simulink model "sm_tVtest_chain_trackSeg"  (R2026a)
settings: Solver=ode23t  AbsTol=1e-3  EnableMultiTasking=on
undefined symbols (not defined in the file): Excv, ExcvI2R4, X, Y, Z
libraries: sm_lib x13, sm_trackV_lib_chain_segment x12, nesl_utility x1
Description:
  | Excavator Track Segments
  | Copyright 2023-2026 The MathWorks, Inc.
settings Model: Creator=smiller  LastModifiedBy=smiller
settings DebuggingCC: SubsystemReferenceDiagnosticForUnitTest=warning
settings SimscapeCC: SimscapeNominalValues="[{\"value\":\"1\",\"unit\":\"A\"},{\"value\":\"1\",\"unit\":\"bar\"},{\"value\":\"1\",\"unit\":\"cm^2\"},{\"value\":\"1\",\"unit\":\"cm^3/s\"},{\"value\":\"1\",\"unit\":\"kJ/kg\"},{\"value\":\"1\",\"unit\":\"kW\"},{\"value\":\"1\",\"unit\":\"l\"},{\"value\":\"1\",\"unit\":\"N\"},{\"value\":\"1\",\"unit\":\"N*m\"},{\"value\":\"1\",\"unit\":\"V\"}]"  SimscapeLogSimulationStatistics=on
settings ExplorerConfigSet: InternalSimMechanicsExplorerSettings="<ExplorerConfiguration><canonicalview>default</canonicalview><AnimationSetting><BasePlaybackSpeed>1.0</BasePlaybackSpeed><PlaybackSpeedFactor>1.0</PlaybackSpeedFactor></AnimationSetting><TilePanel><TileInfo><Tiles Columns=\"1\" Count=\"1\" Rows=\"1\"><Column Weight=\"1\"/><Row Weight=\"1\"/><Tile Height=\"1\" Width=\"1\" X=\"0\" Y=\"0\"/></Tiles></TileInfo><SceneInfo><SceneViewer><BGColor><R>1</R><G>1</G><B>1</B></BGColor><Camera><DoPerspective>off</DoPerspective><Position><X>0.602162155298437085</X><Y>-1.48336517440419313</Y><Z>-12.2297850923587443</Z></Position><Center><X>-0.207049076284216343</X><Y>-0.366682176808429294</Y><Z>0.0032695390144664941</Z></Center><Up><X>0.00405979016857013243</X><Y>0.995875537710112058</Y><Z>-0.0906390175056120545</Z></Up><ViewLimDist>1</ViewLimDist><YLim>0.528639925542969458</YLim><XLim>0.496349528694795095</XLim></Camera></SceneViewer></SceneInfo></TilePanel><MechEditorPanel><Cameras/><GfxPanelCameraMap/><VideoCreator><PlaybackSpeedRatio>1.0</PlaybackSpeedRatio><FrameRate>30</FrameRate><VideoFormat>Motion JPEG AVI</VideoFormat><FrameSize>auto</FrameSize></VideoCreator></MechEditorPanel></ExplorerConfiguration>"

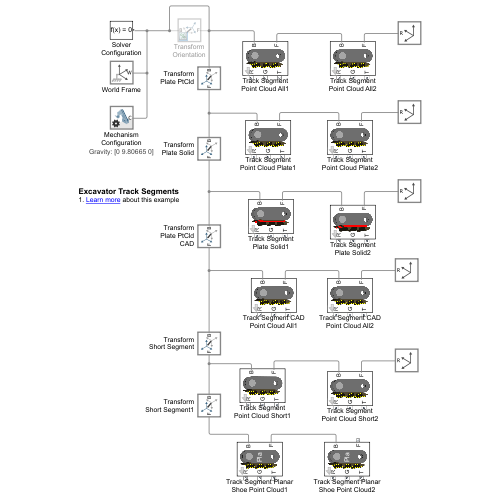
[thumbnail: Simulink's stored preview of the top-level diagram]
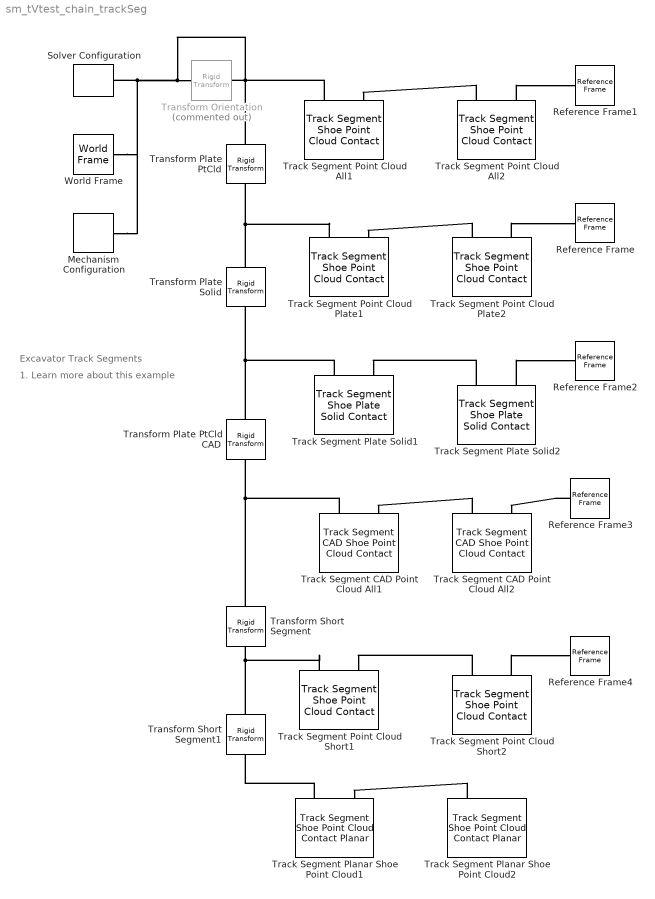
== system sm_tVtest_chain_trackSeg ==
  note: Excavator Track Segments
  note: 1. Learn more about this example
  Mechanism Configuration : sm_lib/Utilities/Mechanism Configuration  UniformGravity=Constant  GravityVector=[0 9.80665 0]  GravityVectorUnits=m/s^2  LinearizationDelta=0.001  JointModeTransitionNonlinearIterations=2
      settings: AttributesFormatString=Gravity: %<GravityVector>
  Reference Frame{,1..4} (5 alike) : sm_lib/Frames and Transforms/Reference Frame
  Solver Configuration : nesl_utility/Solver Configuration  PhysicalDomain=network_engine_domain  SubClassName=solver  LeftPortType=input  RightPortType=generic  Tones=[]  Harmonics=[]  SimulateNoise=off  Profile=off  UseLocalSampling=off  EnableSwitchedLinearOptims=on  FrequencyDomain=off  UseCCode=off  RelTol=0.001  AbsTol=1e-06  MinStep=1e-09  ToWorkspace=off  RevertToSquareIcSolve=off  NumHomotopyIterations=100  PhasorMode=off  PhasorModeNumHarmonics=1  ConsistencySolver=NEWTON_XTOL_AFTER_FTOL  CanonicalOrdering=UNORDERED  OptimizeIntermediates=UNOPTIMIZED  IndexReductionMethod=DerivativeReplacement  DoDC=off  ResidualTolerance=1e-09  ConsistencyTolSource=GLOBAL  ConsistencyAbsTol=0.001  ConsistencyRelTol=0.001  ConsistencyTolFactor=0.001  UseLocalSolver=off  LocalSolverChoice=NE_BACKWARD_EULER_ADVANCER  ResolveIndetEquations=on  FunctionEvalNumThread=1  LocalSolverSampleTime=0.001  DoFixedCost=off  MaxNonlinIter=3  MaxModeIter=2  ComputeImpulses=off  ImpulseIterations=2  LinearAlgebra=Sparse  LinearAlgebraNumThread=0  EquationFormulation=NE_TIME_EF  DelaysMemoryBudget=1024  AutomaticFiltering=on  FilteringTimeConstant=0.001  PartitionStorageMethod=AS_NEEDED  PartitionMemoryBudget=1024  PartitionMethod=FAST  MultibodyUseLocalSolver=off  MultibodyLocalSolverChoice=ODE1  MultibodyLocalSolverSampleTime=0.001
  Track Segment Plate Solid1 : sm_trackV_lib_chain_segment/Track Segment Shoe Plate Solid Contact  chain_wid=Excv.Chain.chain_wid  chain_seg_m=Excv.Chain.link_m  chain_seg_cg=Excv.Chain.link_cg  chain_seg_moi=Excv.Chain.link_moi  chain_seg_poi=Excv.Chain.link_poi  plate_h=Excv.Chain.plate_h  plate_xc=Excv.Chain.plate_xc  plate_thk=Excv.Chain.plate_thk  pin_sep=Excv.Chain.pin_sep  plate_ang=Excv.Chain.plate_ang  plate_clr=Excv.Chain.plate_clr  plate_opc=Excv.Chain.plate_opc  pin_len=Excv.Chain.pin_len  pin_rad=Excv.Chain.pin_rad  pin_clr=Excv.Chain.pin_clr  pin_opc=Excv.Chain.pin_opc  shoe_xc=Excv.Shoe.xc  shoe_w=Excv.Shoe.w  shoe_m=Excv.Shoe.mass  shoe_cg=Excv.Shoe.cg  shoe_moi=Excv.Shoe.moi  shoe_poi=Excv.Shoe.poi  shoe_clr=Excv.Shoe.clr  shoe_opc=Excv.Shoe.opc  posTgtSpecify=on  posTgtPriority=High  PositionTargetValue=0  DampingCoefficient=1.0  shoe_plate_h=Excv.Shoe.pad_h  shoe_plate_l=Excv.Shoe.l  shoe_plate_contact_clr=Excv.Shoe.ground_contact.plate_solid.clr  shoe_plate_contact_opc=Excv.Shoe.ground_contact.plate_solid.opc*0+1  chain_to_roller_clr=Excv.Chain.roller_contact.clr  chain_to_roller_opc=Excv.Chain.roller_contact.opc  chain_to_teeth_clr=Excv.Chain.teeth_contact.clr  chain_to_teeth_opc=Excv.Chain.teeth_contact.opc
  Track Segment Plate Solid2 : sm_trackV_lib_chain_segment/Track Segment Shoe Plate Solid Contact  chain_wid=Excv.Chain.chain_wid  chain_seg_m=Excv.Chain.link_m  chain_seg_cg=Excv.Chain.link_cg  chain_seg_moi=Excv.Chain.link_moi  chain_seg_poi=Excv.Chain.link_poi  plate_h=Excv.Chain.plate_h  plate_xc=Excv.Chain.plate_xc  plate_thk=Excv.Chain.plate_thk  pin_sep=Excv.Chain.pin_sep  plate_ang=Excv.Chain.plate_ang  plate_clr=Excv.Chain.plate_clr  plate_opc=Excv.Chain.plate_opc  pin_len=Excv.Chain.pin_len  pin_rad=Excv.Chain.pin_rad  pin_clr=Excv.Chain.pin_clr  pin_opc=Excv.Chain.pin_opc  shoe_xc=Excv.Shoe.xc  shoe_w=Excv.Shoe.w  shoe_m=Excv.Shoe.mass  shoe_cg=Excv.Shoe.cg  shoe_moi=Excv.Shoe.moi  shoe_poi=Excv.Shoe.poi  shoe_clr=Excv.Shoe.clr  shoe_opc=Excv.Shoe.opc  posTgtSpecify=on  posTgtPriority=High  PositionTargetValue=0  DampingCoefficient=1.0  shoe_plate_h=Excv.Shoe.pad_h  shoe_plate_l=Excv.Shoe.l  shoe_plate_contact_clr=Excv.Shoe.ground_contact.plate_solid.clr  shoe_plate_contact_opc=Excv.Shoe.ground_contact.plate_solid.opc*0+1  chain_to_roller_clr=Excv.Chain.roller_contact.clr  chain_to_roller_opc=Excv.Chain.roller_contact.opc  chain_to_teeth_clr=Excv.Chain.teeth_contact.clr  chain_to_teeth_opc=Excv.Chain.teeth_contact.opc
  Track Segment Point Cloud All1 : sm_trackV_lib_chain_segment/Track Segment Shoe Point Cloud Contact  chain_wid=Excv.Chain.chain_wid  chain_seg_m=Excv.Chain.link_m  chain_seg_cg=Excv.Chain.link_cg  chain_seg_moi=Excv.Chain.link_moi  chain_seg_poi=Excv.Chain.link_poi  plate_h=Excv.Chain.plate_h  plate_xc=Excv.Chain.plate_xc  plate_thk=Excv.Chain.plate_thk  pin_sep=Excv.Chain.pin_sep  plate_ang=Excv.Chain.plate_ang  plate_clr=Excv.Chain.plate_clr  plate_opc=Excv.Chain.plate_opc  pin_len=Excv.Chain.pin_len  pin_rad=Excv.Chain.pin_rad  pin_clr=Excv.Chain.pin_clr  pin_opc=Excv.Chain.pin_opc  shoe_xc=Excv.Shoe.xc  shoe_w=Excv.Shoe.w  shoe_m=Excv.Shoe.mass  shoe_cg=Excv.Shoe.cg  shoe_moi=Excv.Shoe.moi  shoe_poi=Excv.Shoe.poi  shoe_clr=Excv.Shoe.clr  shoe_opc=Excv.Shoe.opc  posTgtSpecify=on  posTgtPriority=High  PositionTargetValue=0  DampingCoefficient=1.0  ptcld_shoe=[Excv.Shoe.ptcld_sets.plate;Excv.Shoe.ptcld_sets.grousers]  ptcld_shoe_rad=Excv.Shoe.ground_contact.ptcld.rad  ptcld_shoe_clr=Excv.Shoe.ground_contact.ptcld.clr  ptcld_shoe_opc=Excv.Shoe.ground_contact.ptcld.opc  chain_to_roller_clr=Excv.Chain.roller_contact.clr  chain_to_roller_opc=Excv.Chain.roller_contact.opc  chain_to_teeth_clr=Excv.Chain.teeth_contact.clr  chain_to_teeth_opc=Excv.Chain.teeth_contact.opc
  Track Segment Point Cloud All2 : sm_trackV_lib_chain_segment/Track Segment Shoe Point Cloud Contact  chain_wid=Excv.Chain.chain_wid  chain_seg_m=Excv.Chain.link_m  chain_seg_cg=Excv.Chain.link_cg  chain_seg_moi=Excv.Chain.link_moi  chain_seg_poi=Excv.Chain.link_poi  plate_h=Excv.Chain.plate_h  plate_xc=Excv.Chain.plate_xc  plate_thk=Excv.Chain.plate_thk  pin_sep=Excv.Chain.pin_sep  plate_ang=Excv.Chain.plate_ang  plate_clr=Excv.Chain.plate_clr  plate_opc=Excv.Chain.plate_opc  pin_len=Excv.Chain.pin_len  pin_rad=Excv.Chain.pin_rad  pin_clr=Excv.Chain.pin_clr  pin_opc=Excv.Chain.pin_opc  shoe_xc=Excv.Shoe.xc  shoe_w=Excv.Shoe.w  shoe_m=Excv.Shoe.mass  shoe_cg=Excv.Shoe.cg  shoe_moi=Excv.Shoe.moi  shoe_poi=Excv.Shoe.poi  shoe_clr=Excv.Shoe.clr  shoe_opc=Excv.Shoe.opc  posTgtSpecify=on  posTgtPriority=High  PositionTargetValue=0  DampingCoefficient=1.0  ptcld_shoe=[Excv.Shoe.ptcld_sets.plate;Excv.Shoe.ptcld_sets.grousers]  ptcld_shoe_rad=Excv.Shoe.ground_contact.ptcld.rad  ptcld_shoe_clr=Excv.Shoe.ground_contact.ptcld.clr  ptcld_shoe_opc=Excv.Shoe.ground_contact.ptcld.opc  chain_to_roller_clr=Excv.Chain.roller_contact.clr  chain_to_roller_opc=Excv.Chain.roller_contact.opc+0.5  chain_to_teeth_clr=Excv.Chain.teeth_contact.clr  chain_to_teeth_opc=Excv.Chain.teeth_contact.opc
  Track Segment Point Cloud Plate1 : sm_trackV_lib_chain_segment/Track Segment Shoe Point Cloud Contact  chain_wid=Excv.Chain.chain_wid  chain_seg_m=Excv.Chain.link_m  chain_seg_cg=Excv.Chain.link_cg  chain_seg_moi=Excv.Chain.link_moi  chain_seg_poi=Excv.Chain.link_poi  plate_h=Excv.Chain.plate_h  plate_xc=Excv.Chain.plate_xc  plate_thk=Excv.Chain.plate_thk  pin_sep=Excv.Chain.pin_sep  plate_ang=Excv.Chain.plate_ang  plate_clr=Excv.Chain.plate_clr  plate_opc=Excv.Chain.plate_opc  pin_len=Excv.Chain.pin_len  pin_rad=Excv.Chain.pin_rad  pin_clr=Excv.Chain.pin_clr  pin_opc=Excv.Chain.pin_opc  shoe_xc=Excv.Shoe.xc  shoe_w=Excv.Shoe.w  shoe_m=Excv.Shoe.mass  shoe_cg=Excv.Shoe.cg  shoe_moi=Excv.Shoe.moi  shoe_poi=Excv.Shoe.poi  shoe_clr=Excv.Shoe.clr  shoe_opc=Excv.Shoe.opc  posTgtSpecify=on  posTgtPriority=High  PositionTargetValue=0  DampingCoefficient=1.0  ptcld_shoe=Excv.Shoe.ptcld_sets.plate  ptcld_shoe_rad=Excv.Shoe.ground_contact.ptcld.rad  ptcld_shoe_clr=Excv.Shoe.ground_contact.ptcld.clr  ptcld_shoe_opc=Excv.Shoe.ground_contact.ptcld.opc  chain_to_roller_clr=Excv.Chain.roller_contact.clr  chain_to_roller_opc=Excv.Chain.roller_contact.opc  chain_to_teeth_clr=Excv.Chain.teeth_contact.clr  chain_to_teeth_opc=Excv.Chain.teeth_contact.opc
  Track Segment Point Cloud Plate2 : sm_trackV_lib_chain_segment/Track Segment Shoe Point Cloud Contact  chain_wid=Excv.Chain.chain_wid  chain_seg_m=Excv.Chain.link_m  chain_seg_cg=Excv.Chain.link_cg  chain_seg_moi=Excv.Chain.link_moi  chain_seg_poi=Excv.Chain.link_poi  plate_h=Excv.Chain.plate_h  plate_xc=Excv.Chain.plate_xc  plate_thk=Excv.Chain.plate_thk  pin_sep=Excv.Chain.pin_sep  plate_ang=Excv.Chain.plate_ang  plate_clr=Excv.Chain.plate_clr  plate_opc=Excv.Chain.plate_opc  pin_len=Excv.Chain.pin_len  pin_rad=Excv.Chain.pin_rad  pin_clr=Excv.Chain.pin_clr  pin_opc=Excv.Chain.pin_opc  shoe_xc=Excv.Shoe.xc  shoe_w=Excv.Shoe.w  shoe_m=Excv.Shoe.mass  shoe_cg=Excv.Shoe.cg  shoe_moi=Excv.Shoe.moi  shoe_poi=Excv.Shoe.poi  shoe_clr=Excv.Shoe.clr  shoe_opc=Excv.Shoe.opc  posTgtSpecify=on  posTgtPriority=High  PositionTargetValue=0  DampingCoefficient=1.0  ptcld_shoe=Excv.Shoe.ptcld_sets.plate  ptcld_shoe_rad=Excv.Shoe.ground_contact.ptcld.rad  ptcld_shoe_clr=Excv.Shoe.ground_contact.ptcld.clr  ptcld_shoe_opc=Excv.Shoe.ground_contact.ptcld.opc  chain_to_roller_clr=Excv.Chain.roller_contact.clr  chain_to_roller_opc=Excv.Chain.roller_contact.opc  chain_to_teeth_clr=Excv.Chain.teeth_contact.clr  chain_to_teeth_opc=Excv.Chain.teeth_contact.opc
  Track Segment Point Cloud Short1 : sm_trackV_lib_chain_segment/Track Segment Shoe Point Cloud Contact  chain_wid=ExcvI2R4.Chain.chain_wid  chain_seg_m=ExcvI2R4.Chain.link_m  chain_seg_cg=ExcvI2R4.Chain.link_cg  chain_seg_moi=ExcvI2R4.Chain.link_moi  chain_seg_poi=ExcvI2R4.Chain.link_poi  plate_h=ExcvI2R4.Chain.plate_h  plate_xc=ExcvI2R4.Chain.plate_xc  plate_thk=ExcvI2R4.Chain.plate_thk  pin_sep=ExcvI2R4.Chain.pin_sep  plate_ang=ExcvI2R4.Chain.plate_ang  plate_clr=ExcvI2R4.Chain.plate_clr  plate_opc=ExcvI2R4.Chain.plate_opc  pin_len=ExcvI2R4.Chain.pin_len  pin_rad=ExcvI2R4.Chain.pin_rad  pin_clr=ExcvI2R4.Chain.pin_clr  pin_opc=ExcvI2R4.Chain.pin_opc  shoe_xc=ExcvI2R4.Shoe.xc  shoe_w=ExcvI2R4.Shoe.w  shoe_m=ExcvI2R4.Shoe.mass  shoe_cg=ExcvI2R4.Shoe.cg  shoe_moi=ExcvI2R4.Shoe.moi  shoe_poi=ExcvI2R4.Shoe.poi  shoe_clr=ExcvI2R4.Shoe.clr  shoe_opc=ExcvI2R4.Shoe.opc  posTgtSpecify=on  posTgtPriority=High  PositionTargetValue=0  DampingCoefficient=1.0  ptcld_shoe=[ExcvI2R4.Shoe.ptcld_sets.plate;ExcvI2R4.Shoe.ptcld_sets.grousers]  ptcld_shoe_rad=ExcvI2R4.Shoe.ground_contact.ptcld.rad  ptcld_shoe_clr=ExcvI2R4.Shoe.ground_contact.ptcld.clr  ptcld_shoe_opc=ExcvI2R4.Shoe.ground_contact.ptcld.opc  chain_to_roller_clr=ExcvI2R4.Chain.roller_contact.clr  chain_to_roller_opc=ExcvI2R4.Chain.roller_contact.opc  chain_to_teeth_clr=ExcvI2R4.Chain.teeth_contact.clr  chain_to_teeth_opc=ExcvI2R4.Chain.teeth_contact.opc
  Track Segment Point Cloud Short2 : sm_trackV_lib_chain_segment/Track Segment Shoe Point Cloud Contact  chain_wid=ExcvI2R4.Chain.chain_wid  chain_seg_m=ExcvI2R4.Chain.link_m  chain_seg_cg=ExcvI2R4.Chain.link_cg  chain_seg_moi=ExcvI2R4.Chain.link_moi  chain_seg_poi=ExcvI2R4.Chain.link_poi  plate_h=ExcvI2R4.Chain.plate_h  plate_xc=ExcvI2R4.Chain.plate_xc  plate_thk=ExcvI2R4.Chain.plate_thk  pin_sep=ExcvI2R4.Chain.pin_sep  plate_ang=ExcvI2R4.Chain.plate_ang  plate_clr=ExcvI2R4.Chain.plate_clr  plate_opc=ExcvI2R4.Chain.plate_opc  pin_len=ExcvI2R4.Chain.pin_len  pin_rad=ExcvI2R4.Chain.pin_rad  pin_clr=ExcvI2R4.Chain.pin_clr  pin_opc=ExcvI2R4.Chain.pin_opc  shoe_xc=ExcvI2R4.Shoe.xc  shoe_w=ExcvI2R4.Shoe.w  shoe_m=ExcvI2R4.Shoe.mass  shoe_cg=ExcvI2R4.Shoe.cg  shoe_moi=ExcvI2R4.Shoe.moi  shoe_poi=ExcvI2R4.Shoe.poi  shoe_clr=ExcvI2R4.Shoe.clr  shoe_opc=ExcvI2R4.Shoe.opc  posTgtSpecify=on  posTgtPriority=High  PositionTargetValue=0  DampingCoefficient=1.0  ptcld_shoe=[ExcvI2R4.Shoe.ptcld_sets.plate;ExcvI2R4.Shoe.ptcld_sets.grousers]  ptcld_shoe_rad=ExcvI2R4.Shoe.ground_contact.ptcld.rad  ptcld_shoe_clr=ExcvI2R4.Shoe.ground_contact.ptcld.clr  ptcld_shoe_opc=ExcvI2R4.Shoe.ground_contact.ptcld.opc  chain_to_roller_clr=ExcvI2R4.Chain.roller_contact.clr  chain_to_roller_opc=ExcvI2R4.Chain.roller_contact.opc  chain_to_teeth_clr=ExcvI2R4.Chain.teeth_contact.clr  chain_to_teeth_opc=ExcvI2R4.Chain.teeth_contact.opc
  Track Segment CAD Point Cloud All1 : sm_trackV_lib_chain_segment/Track Segment CAD Shoe Point Cloud Contact  chain_wid=Excv.Chain.chain_wid  chain_seg_m=Excv.Chain.link_m  chain_seg_cg=Excv.Chain.link_cg  chain_seg_moi=Excv.Chain.link_moi  chain_seg_poi=Excv.Chain.link_poi  plate_h=Excv.Chain.plate_h  plate_xc=Excv.Chain.plate_xc  plate_thk=Excv.Chain.plate_thk  pin_sep=Excv.Chain.pin_sep  plate_ang=Excv.Chain.plate_ang  plate_clr=Excv.Chain.plate_clr  plate_opc=Excv.Chain.plate_opc  pin_len=Excv.Chain.pin_len  pin_rad=Excv.Chain.pin_rad  pin_clr=Excv.Chain.pin_clr  pin_opc=Excv.Chain.pin_opc  shoe_xc=Excv.Shoe.xc  shoe_w=Excv.Shoe.w  shoe_m=Excv.Shoe.mass  shoe_cg=Excv.Shoe.cg  shoe_moi=Excv.Shoe.moi  shoe_poi=Excv.Shoe.poi  shoe_clr=Excv.Shoe.clr  shoe_opc=Excv.Shoe.opc  posTgtSpecify=on  posTgtPriority=High  PositionTargetValue=0  DampingCoefficient=1.0  ptcld_shoe=[Excv.Shoe.ptcld_sets.cad_plate;Excv.Shoe.ptcld_sets.cad_grousers]  ptcld_shoe_rad=Excv.Shoe.ground_contact.ptcld.rad  ptcld_shoe_clr=Excv.Shoe.ground_contact.ptcld.clr  ptcld_shoe_opc=Excv.Shoe.ground_contact.ptcld.opc  chain_to_roller_clr=Excv.Chain.roller_contact.clr  chain_to_roller_opc=Excv.Chain.roller_contact.opc  chain_to_teeth_clr=Excv.Chain.teeth_contact.clr  chain_to_teeth_opc=Excv.Chain.teeth_contact.opc
  Track Segment CAD Point Cloud All2 : sm_trackV_lib_chain_segment/Track Segment CAD Shoe Point Cloud Contact  chain_wid=Excv.Chain.chain_wid  chain_seg_m=Excv.Chain.link_m  chain_seg_cg=Excv.Chain.link_cg  chain_seg_moi=Excv.Chain.link_moi  chain_seg_poi=Excv.Chain.link_poi  plate_h=Excv.Chain.plate_h  plate_xc=Excv.Chain.plate_xc  plate_thk=Excv.Chain.plate_thk  pin_sep=Excv.Chain.pin_sep  plate_ang=Excv.Chain.plate_ang  plate_clr=Excv.Chain.plate_clr  plate_opc=Excv.Chain.plate_opc  pin_len=Excv.Chain.pin_len  pin_rad=Excv.Chain.pin_rad  pin_clr=Excv.Chain.pin_clr  pin_opc=Excv.Chain.pin_opc  shoe_xc=Excv.Shoe.xc  shoe_w=Excv.Shoe.w  shoe_m=Excv.Shoe.mass  shoe_cg=Excv.Shoe.cg  shoe_moi=Excv.Shoe.moi  shoe_poi=Excv.Shoe.poi  shoe_clr=Excv.Shoe.clr  shoe_opc=Excv.Shoe.opc  posTgtSpecify=on  posTgtPriority=High  PositionTargetValue=0  DampingCoefficient=1.0  ptcld_shoe=[Excv.Shoe.ptcld_sets.cad_plate;Excv.Shoe.ptcld_sets.cad_grousers]  ptcld_shoe_rad=Excv.Shoe.ground_contact.ptcld.rad  ptcld_shoe_clr=Excv.Shoe.ground_contact.ptcld.clr  ptcld_shoe_opc=Excv.Shoe.ground_contact.ptcld.opc  chain_to_roller_clr=Excv.Chain.roller_contact.clr  chain_to_roller_opc=Excv.Chain.roller_contact.opc  chain_to_teeth_clr=Excv.Chain.teeth_contact.clr  chain_to_teeth_opc=Excv.Chain.teeth_contact.opc
  Track Segment Planar Shoe Point Cloud1 : sm_trackV_lib_chain_segment/Track Segment Shoe Point Cloud Contact Planar  chain_wid=Excv.Chain.chain_wid  chain_seg_m=Excv.Chain.link_m  chain_seg_cg=Excv.Chain.link_cg  chain_seg_moi=Excv.Chain.link_moi  chain_seg_poi=Excv.Chain.link_poi  plate_h=Excv.Chain.plate_h  plate_xc=Excv.Chain.plate_xc  plate_thk=Excv.Chain.plate_thk  pin_sep=Excv.Chain.pin_sep  plate_ang=Excv.Chain.plate_ang  plate_clr=Excv.Chain.plate_clr  plate_opc=Excv.Chain.plate_opc*0.2  pin_len=Excv.Chain.pin_len  pin_rad=Excv.Chain.pin_rad  pin_clr=Excv.Chain.pin_clr  pin_opc=Excv.Chain.pin_opc*0.2  shoe_xc=Excv.Shoe.xc  shoe_w=Excv.Shoe.w  shoe_m=Excv.Shoe.mass  shoe_cg=Excv.Shoe.cg  shoe_moi=Excv.Shoe.moi  shoe_poi=Excv.Shoe.poi  shoe_clr=Excv.Shoe.clr  shoe_opc=Excv.Shoe.opc*0.2  posTgtSpecify=on  posTgtPriority=High  PositionTargetValue=0  DampingCoefficient=1.0  ptcld_shoe=Excv.Shoe.ground_contact.ptcld.pts  ptcld_shoe_rad=Excv.Shoe.ground_contact.ptcld.rad  ptcld_shoe_clr=Excv.Shoe.ground_contact.ptcld.clr  ptcld_shoe_opc=Excv.Shoe.ground_contact.ptcld.opc  chain_to_roller_clr=Excv.Chain.roller_contact.clr  chain_to_roller_opc=Excv.Chain.roller_contact.opc+0.5  chain_to_teeth_clr=Excv.Chain.teeth_contact.clr  chain_to_teeth_opc=Excv.Chain.teeth_contact.opc
  Track Segment Planar Shoe Point Cloud2 : sm_trackV_lib_chain_segment/Track Segment Shoe Point Cloud Contact Planar  chain_wid=Excv.Chain.chain_wid  chain_seg_m=Excv.Chain.link_m  chain_seg_cg=Excv.Chain.link_cg  chain_seg_moi=Excv.Chain.link_moi  chain_seg_poi=Excv.Chain.link_poi  plate_h=Excv.Chain.plate_h  plate_xc=Excv.Chain.plate_xc  plate_thk=Excv.Chain.plate_thk  pin_sep=Excv.Chain.pin_sep  plate_ang=Excv.Chain.plate_ang  plate_clr=Excv.Chain.plate_clr  plate_opc=Excv.Chain.plate_opc*0.2  pin_len=Excv.Chain.pin_len  pin_rad=Excv.Chain.pin_rad  pin_clr=Excv.Chain.pin_clr  pin_opc=Excv.Chain.pin_opc*0.2  shoe_xc=Excv.Shoe.xc  shoe_w=Excv.Shoe.w  shoe_m=Excv.Shoe.mass  shoe_cg=Excv.Shoe.cg  shoe_moi=Excv.Shoe.moi  shoe_poi=Excv.Shoe.poi  shoe_clr=Excv.Shoe.clr  shoe_opc=Excv.Shoe.opc*0.2  posTgtSpecify=on  posTgtPriority=High  PositionTargetValue=0  DampingCoefficient=1.0  ptcld_shoe=[Excv.Shoe.ptcld_sets.plate;Excv.Shoe.ptcld_sets.grousers]  ptcld_shoe_rad=Excv.Shoe.ground_contact.ptcld.rad  ptcld_shoe_clr=Excv.Shoe.ground_contact.ptcld.clr  ptcld_shoe_opc=Excv.Shoe.ground_contact.ptcld.opc  chain_to_roller_clr=Excv.Chain.roller_contact.clr  chain_to_roller_opc=Excv.Chain.roller_contact.opc+0.5  chain_to_teeth_clr=Excv.Chain.teeth_contact.clr  chain_to_teeth_opc=Excv.Chain.teeth_contact.opc
  Transform Orientation : sm_lib/Frames and Transforms/Rigid Transform  Commented=on  RotationMethod=StandardAxis  FollAlignAxisA=+X  BaseAlignAxisA=+Y  FollAlignAxisB=+Y  BaseAlignAxisB=+Z  RotationStandardAxis=+X  RotationAngle=90  RotationAngleUnits=deg  RotationArbitraryAxis=[0 0 1]  RotationSequenceAxes=FollowerAxes  RotationSequence=XYX  RotationSequenceAngles=[0 0 0]  RotationSequenceAnglesUnits=deg  RotationMatrix=[1 0 0; 0 1 0; 0 0 1]  Quaternion=[1 0 0 0]  TranslationMethod=None  TranslationCartesianOffset=[0 0 0]  TranslationCartesianOffsetUnits=m  TranslationStandardAxis=+Z  TranslationStandardOffset=0  TranslationStandardOffsetUnits=m  TranslationROffset=0  TranslationROffsetUnits=m  TranslationThetaOffset=0  TranslationThetaOffsetUnits=deg  TranslationZOffset=0  TranslationZOffsetUnits=m
  Transform Plate PtCld : sm_lib/Frames and Transforms/Rigid Transform  RotationMethod=None  FollAlignAxisA=+X  BaseAlignAxisA=+Y  FollAlignAxisB=+Y  BaseAlignAxisB=+Z  RotationStandardAxis=+X  RotationAngle=90  RotationAngleUnits=deg  RotationArbitraryAxis=[0 0 1]  RotationSequenceAxes=FollowerAxes  RotationSequence=XYX  RotationSequenceAngles=[0 0 0]  RotationSequenceAnglesUnits=deg  RotationMatrix=[1 0 0; 0 1 0; 0 0 1]  Quaternion=[1 0 0 0]  TranslationMethod=StandardAxis  TranslationCartesianOffset=[0 0 0]  TranslationCartesianOffsetUnits=m  TranslationStandardAxis=-Y  TranslationStandardOffset=0.25  TranslationStandardOffsetUnits=m  TranslationROffset=0  TranslationROffsetUnits=m  TranslationThetaOffset=0  TranslationThetaOffsetUnits=deg  TranslationZOffset=0  TranslationZOffsetUnits=m
  Transform Plate PtCld CAD : sm_lib/Frames and Transforms/Rigid Transform  RotationMethod=None  FollAlignAxisA=+X  BaseAlignAxisA=+Y  FollAlignAxisB=+Y  BaseAlignAxisB=+Z  RotationStandardAxis=+X  RotationAngle=90  RotationAngleUnits=deg  RotationArbitraryAxis=[0 0 1]  RotationSequenceAxes=FollowerAxes  RotationSequence=XYX  RotationSequenceAngles=[0 0 0]  RotationSequenceAnglesUnits=deg  RotationMatrix=[1 0 0; 0 1 0; 0 0 1]  Quaternion=[1 0 0 0]  TranslationMethod=StandardAxis  TranslationCartesianOffset=[0 0 0]  TranslationCartesianOffsetUnits=m  TranslationStandardAxis=-Y  TranslationStandardOffset=0.25  TranslationStandardOffsetUnits=m  TranslationROffset=0  TranslationROffsetUnits=m  TranslationThetaOffset=0  TranslationThetaOffsetUnits=deg  TranslationZOffset=0  TranslationZOffsetUnits=m
  Transform Plate Solid : sm_lib/Frames and Transforms/Rigid Transform  RotationMethod=None  FollAlignAxisA=+X  BaseAlignAxisA=+Y  FollAlignAxisB=+Y  BaseAlignAxisB=+Z  RotationStandardAxis=+X  RotationAngle=90  RotationAngleUnits=deg  RotationArbitraryAxis=[0 0 1]  RotationSequenceAxes=FollowerAxes  RotationSequence=XYX  RotationSequenceAngles=[0 0 0]  RotationSequenceAnglesUnits=deg  RotationMatrix=[1 0 0; 0 1 0; 0 0 1]  Quaternion=[1 0 0 0]  TranslationMethod=StandardAxis  TranslationCartesianOffset=[0 0 0]  TranslationCartesianOffsetUnits=m  TranslationStandardAxis=-Y  TranslationStandardOffset=0.25  TranslationStandardOffsetUnits=m  TranslationROffset=0  TranslationROffsetUnits=m  TranslationThetaOffset=0  TranslationThetaOffsetUnits=deg  TranslationZOffset=0  TranslationZOffsetUnits=m
  Transform Short Segment : sm_lib/Frames and Transforms/Rigid Transform  RotationMethod=None  FollAlignAxisA=+X  BaseAlignAxisA=+Y  FollAlignAxisB=+Y  BaseAlignAxisB=+Z  RotationStandardAxis=+X  RotationAngle=90  RotationAngleUnits=deg  RotationArbitraryAxis=[0 0 1]  RotationSequenceAxes=FollowerAxes  RotationSequence=XYX  RotationSequenceAngles=[0 0 0]  RotationSequenceAnglesUnits=deg  RotationMatrix=[1 0 0; 0 1 0; 0 0 1]  Quaternion=[1 0 0 0]  TranslationMethod=StandardAxis  TranslationCartesianOffset=[0 0 0]  TranslationCartesianOffsetUnits=m  TranslationStandardAxis=-Y  TranslationStandardOffset=0.25  TranslationStandardOffsetUnits=m  TranslationROffset=0  TranslationROffsetUnits=m  TranslationThetaOffset=0  TranslationThetaOffsetUnits=deg  TranslationZOffset=0  TranslationZOffsetUnits=m
  Transform Short Segment1 : sm_lib/Frames and Transforms/Rigid Transform  RotationMethod=None  FollAlignAxisA=+X  BaseAlignAxisA=+Y  FollAlignAxisB=+Y  BaseAlignAxisB=+Z  RotationStandardAxis=+X  RotationAngle=90  RotationAngleUnits=deg  RotationArbitraryAxis=[0 0 1]  RotationSequenceAxes=FollowerAxes  RotationSequence=XYX  RotationSequenceAngles=[0 0 0]  RotationSequenceAnglesUnits=deg  RotationMatrix=[1 0 0; 0 1 0; 0 0 1]  Quaternion=[1 0 0 0]  TranslationMethod=StandardAxis  TranslationCartesianOffset=[0 0 0]  TranslationCartesianOffsetUnits=m  TranslationStandardAxis=-Y  TranslationStandardOffset=0.25  TranslationStandardOffsetUnits=m  TranslationROffset=0  TranslationROffsetUnits=m  TranslationThetaOffset=0  TranslationThetaOffsetUnits=deg  TranslationZOffset=0  TranslationZOffsetUnits=m
  World Frame : sm_lib/Frames and Transforms/World Frame
  connections:
  Transform Plate PtCld/LConn1 -- Track Segment Point Cloud All1/LConn1 -- Transform Orientation/LConn1 -- World Frame/RConn1 -- Mechanism Configuration/RConn1 -- Solver Configuration/RConn1 -- Transform Orientation/RConn1
  Track Segment Point Cloud All2/LConn1 -- Track Segment Point Cloud All1/LConn2
  Track Segment Point Cloud Plate1/LConn1 -- Transform Plate PtCld/RConn1 -- Transform Plate Solid/LConn1
  Track Segment Point Cloud Plate2/LConn1 -- Track Segment Point Cloud Plate1/LConn2
  Track Segment Point Cloud All2/LConn2 -- Reference Frame1/RConn1
  Track Segment Point Cloud Plate2/LConn2 -- Reference Frame/RConn1
  Track Segment Plate Solid1/LConn1 -- Transform Plate PtCld CAD/LConn1 -- Transform Plate Solid/RConn1
  Track Segment Plate Solid2/LConn1 -- Track Segment Plate Solid1/LConn2
  Track Segment Plate Solid2/LConn2 -- Reference Frame2/RConn1
  Track Segment CAD Point Cloud All1/LConn1 -- Transform Plate PtCld CAD/RConn1 -- Transform Short Segment/LConn1
  Track Segment CAD Point Cloud All2/LConn1 -- Track Segment CAD Point Cloud All1/LConn2
  Reference Frame3/RConn1 -- Track Segment CAD Point Cloud All2/LConn2
  Track Segment Point Cloud Short2/LConn1 -- Track Segment Point Cloud Short1/LConn2
  Track Segment Point Cloud Short2/LConn2 -- Reference Frame4/RConn1
  Track Segment Point Cloud Short1/LConn1 -- Transform Short Segment1/LConn1 -- Transform Short Segment/RConn1
  Track Segment Planar Shoe Point Cloud1/LConn1 -- Transform Short Segment1/RConn1
  Track Segment Planar Shoe Point Cloud2/LConn1 -- Track Segment Planar Shoe Point Cloud1/LConn2
